simulink model "lab5_model"  (R2018a)
settings: Solver=ode5  StartTime=0.0  StopTime=5*140*0.75  RelTol=1e-3  EnableMultiTasking=on
values from neighbouring files (symbols this model uses):
  C_obsrv = H'    [lab5.m]    (also in matlab.mat = [0 1])
  G_obsrv = G'    [lab5.m]    (also in matlab.mat = [0  -0.0930764048847; 1  1.06683801313])
  H_obsrv = C'    [lab5.m]    (also in matlab.mat = [0.053077183427 0.0186922775571])
libraries: simulink x2
settings Model: Creator=My Project  LastModifiedBy=jasonchen
settings DataIOCC: LimitDataPoints=on
settings OptimizationCC: LifeSpan=inf
settings DebuggingCC: AllowSymbolicDim=off  SFUnexpectedBacktrackingDiag=warning  SFNoUnconditionalDefaultTransitionDiag=warning  SFExecutionAtInitializationDiag=none
settings HardwareCC: ProdBitPerLong=64  ProdLargestAtomicFloat=None  ProdHWDeviceType=Intel->x86-64  TargetBitPerLong=64  TargetBitPerPointer=64  TargetIntDivRoundTo=Zero  TargetEndianess=LittleEndian  TargetWordSize=64  TargetHWDeviceType=Intel->x86-64
settings ModelReferenceCC: PropagateSignalLabelsOutOfModel=off
settings RTWCC: SystemTargetFile=sldrt.tlc  TemplateMakefile=sldrt.tmf  Description=Simulink Desktop Real-Time  RTWCompilerOptimization=on
settings CodeAppCC: MaxIdLength=95  StateflowObjectComments=on
settings TargetCC: TargetPreCompLibLocation=C:\Program Files\MATLAB\R2015b\toolbox\sldrt\lib\win64  GeneratePreprocessorConditionals=Use local settings
settings ConfigComp: CovMetricSettings=dw  CovHtmlReporting=on  CovSaveCumulativeToWorkspaceVar=on  CovSaveSingleToWorkspaceVar=on  CovExternalEMLEnable=off

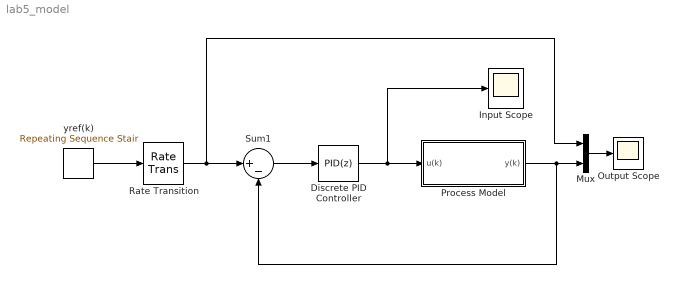
== system lab5_model ==
  Discrete PID Controller : simulink/Continuous/PID Controller  Controller=PID  TimeDomain=Discrete-time  SampleTime=0.75  IntegratorMethod=Forward Euler  FilterMethod=Forward Euler  Form=Parallel  UseFilter=on  ControllerParametersSource=internal  P=0.5  I=0.02  D=0  N=100  InitialConditionSource=internal  InitialConditionForIntegrator=0  InitialConditionForFilter=0  ExternalReset=none  LimitOutput=off  UpperSaturationLimit=inf  LowerSaturationLimit=-inf  LinearizeAsGain=off  AntiWindupMode=none  Kb=1  TrackingMode=off  Kt=1  PParamMin=[]  PParamMax=[]  IParamMin=[]  IParamMax=[]  DParamMin=[]  DParamMax=[]  NParamMin=[]  NParamMax=[]  KbParamMin=[]  KbParamMax=[]  KtParamMin=[]  KtParamMax=[]  POutMin=[]  POutMax=[]  IOutMin=[]  IOutMax=[]  DOutMin=[]  DOutMax=[]  NOutMin=[]  NOutMax=[]  KbOutMin=[]  KbOutMax=[]  KtOutMin=[]  KtOutMax=[]  IntegratorOutMin=[]  IntegratorOutMax=[]  FilterOutMin=[]  FilterOutMax=[]  SumOutMin=[]  SumOutMax=[]  SumI1OutMin=[]  SumI1OutMax=[]  SumI2OutMin=[]  SumI2OutMax=[]  SumI3OutMin=[]  SumI3OutMax=[]  SumDOutMin=[]  SumDOutMax=[]  SaturationOutMin=[]  SaturationOutMax=[]  IntegratorContinuousStateAttributes=''  IntegratorStateMustResolveToSignalObject=off  IntegratorRTWStateStorageClass=Auto  FilterContinuousStateAttributes=''  FilterStateMustResolveToSignalObject=off  FilterRTWStateStorageClass=Auto  DifferentiatorICPrevScaledInput=0  DifferentiatorOutMin=[]  DifferentiatorOutMax=[]  FilterDiffOutCoefMin=[]  FilterDiffOutCoefMax=[]  SumDenOutMin=[]  SumDenOutMax=[]  SumNumOutMin=[]  SumNumOutMax=[]  ReciprocalOutMin=[]  ReciprocalOutMax=[]  DivideOutMin=[]  DivideOutMax=[]  TunerSelectOption=Transfer Function Based (PID Tuner App)
  Input Scope : Scope
  Mux : Mux  Inputs=2
  Output Scope : Scope
  Process Model : Subsystem
  Rate Transition : RateTransition
  Sum1 : Sum  Inputs=|+-
  "yref(k) " : simulink/Sources/Repeating Sequence Stair  OutValues=[0.7 0.2 -0.5 0].'  tsamp=140*0.75  OutMin=[]  OutMax=[]  OutDataTypeStr=double  OutputDataTypeScalingMode=double  OutDataType=fixdt(0,8)  ConRadixGroup=Best Precision: Vector-wise  OutScaling=2^-12
  wires:
  "yref(k) "/1 -> Rate Transition/1
  Mux/1 -> Output Scope/1
  Rate Transition/1 -> Mux/1, Sum1/1
  Sum1/1 -> Discrete PID Controller/1
  Discrete PID Controller/1 -> Process Model/1(u(k)), Input Scope/1
  Process Model/1(y(k)) -> Mux/2, Sum1/2

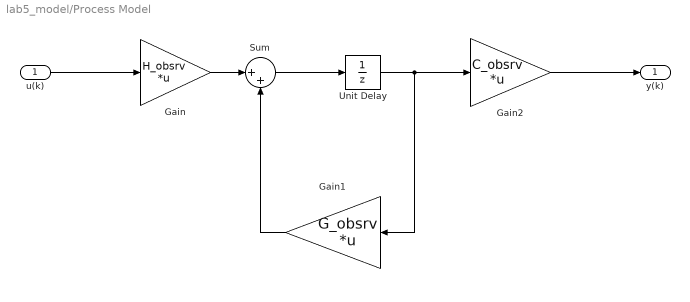
== system lab5_model/Process Model ==
  u(k) : Inport
  Gain : Gain  Gain=H_obsrv  Multiplication=Matrix(K*u)
  Gain1 : Gain  Gain=G_obsrv  Multiplication=Matrix(K*u)
  Gain2 : Gain  Gain=C_obsrv  Multiplication=Matrix(K*u)
  Sum : Sum  Inputs=|++
  Unit Delay : UnitDelay  SampleTime=0.75
  y(k) : Outport
  wires:
  Gain/1 -> Sum/1
  Unit Delay/1 -> Gain1/1, Gain2/1
  Sum/1 -> Unit Delay/1
  Gain1/1 -> Sum/2
  u(k)/1 -> Gain/1
  Gain2/1 -> y(k)/1
